simulink subsystem "LpBiquadFilter"  (R2024a)
settings: Solver=VariableStepAuto  StartTime=0.0  StopTime=10.0  RelTol=1e-3
undefined symbols (not defined in the file or in its folder): vmax, vmin
settings Model: Creator=dfurodet  LastModifiedBy=dfurodet

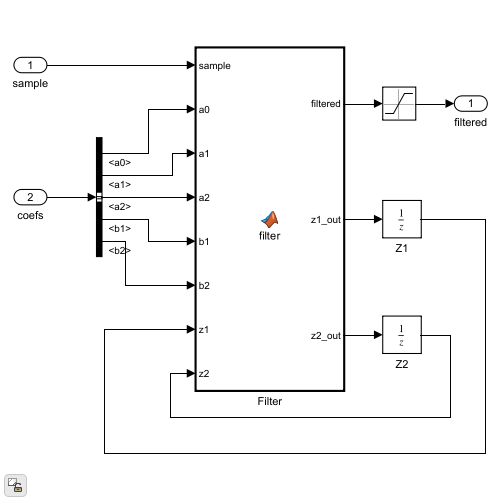
[thumbnail: Simulink's stored preview of the top-level diagram]
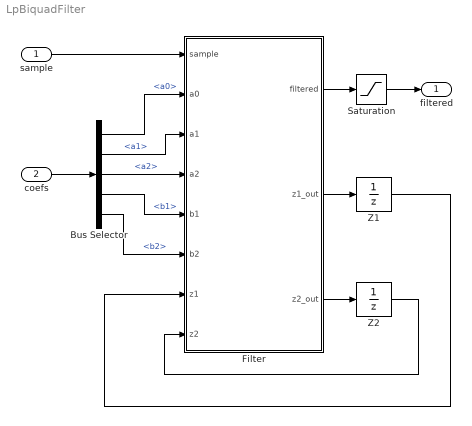
== system LpBiquadFilter ==
  sample : Inport
  coefs : Inport  Port=2
  Bus Selector : BusSelector  OutputSignals=a0,a1,a2,b1,b2
  Filter : MATLAB Function  TreatAsAtomicUnit=on
  Saturation : Saturate  UpperLimit=vmax  LowerLimit=vmin
  Z1 : UnitDelay  SampleTime=-1  HasFrameUpgradeWarning=on
  Z2 : UnitDelay  SampleTime=-1  HasFrameUpgradeWarning=on
  filtered : Outport
  wires:
  Filter/3(z2_out) -> Z2/1
  Filter/1(filtered) -> Saturation/1
  Filter/2(z1_out) -> Z1/1
  Z2/1 -> Filter/8(z2)
  Z1/1 -> Filter/7(z1)
  sample/1 -> Filter/1(sample)
  Saturation/1 -> filtered/1
  coefs/1 -> Bus Selector/1
  Bus Selector/1 -> Filter/2(a0)  "<a0>"
  Bus Selector/2 -> Filter/3(a1)  "<a1>"
  Bus Selector/3 -> Filter/4(a2)  "<a2>"
  Bus Selector/4 -> Filter/5(b1)  "<b1>"
  Bus Selector/5 -> Filter/6(b2)  "<b2>"

== matlab function LpBiquadFilter/Filter ==
  data: sample input; filtered output; a0 input; a1 input; a2 input; b1 input; b2 input; z1 input single; z2 input single; z1_out output; z2_out output
function [filtered, z1_out, z2_out] = filter(sample, a0, a1, a2, b1, b2, z1, z2)
    filtered = a0 * sample + z1;
    z1_out = a1 * sample + z2 - b1 * filtered;
    z2_out = a2 * sample - b2 * filtered;
end
